simulink model "may21_slk"  (R2023b)
settings: Solver=VariableStepAuto  StartTime=0.0  StopTime=Tend_slk  RelTol=1e-3
values from neighbouring files (symbols this model uses):
  Ts_slk = 0.01    [may21_b_ml.m]    (also in may21_ml.m)
libraries: cstblocks x4, simulink x2
settings Model: Creator=Camilla  LastModifiedBy=Camilla

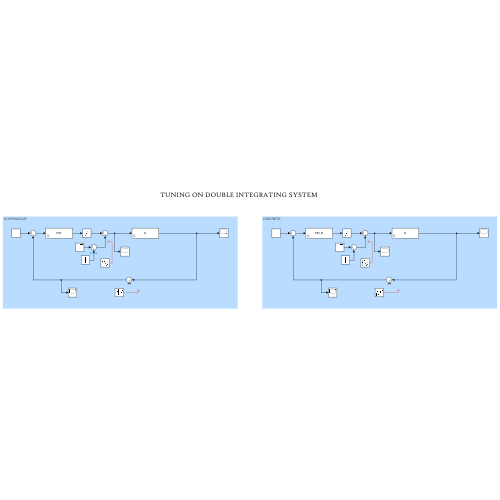
[thumbnail: Simulink's stored preview of the top-level diagram]
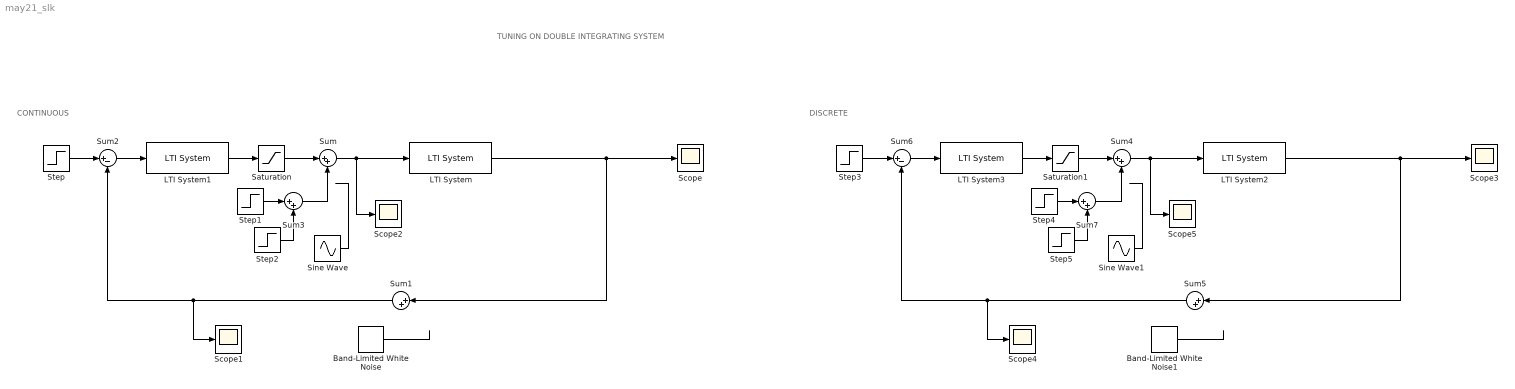
== system may21_slk ==
  note: TUNING ON DOUBLE INTEGRATING SYSTEM
  note: CONTINUOUS
  note: DISCRETE
  Band-Limited White Noise : simulink/Sources/Band-Limited White Noise  Cov=[0.0001]  Ts=0.05  seed=[23341]
  Band-Limited White Noise1 : simulink/Sources/Band-Limited White Noise  Cov=[0.0001]  Ts=0.05  seed=[23341]
  LTI System : cstblocks/LTI System  sys=G  IC=[]  PadeOrder=0
  LTI System1 : cstblocks/LTI System  sys=PID  IC=[]  PadeOrder=0
  LTI System2 : cstblocks/LTI System  sys=G  IC=[]  PadeOrder=0
  LTI System3 : cstblocks/LTI System  sys=PID_D  IC=[]  PadeOrder=0
  Saturation : Saturate  UpperLimit=1.2  LowerLimit=-1.2
  Saturation1 : Saturate  UpperLimit=1.2  LowerLimit=-1.2
  Scope{,1..5} (6 alike) : Scope
  Sine Wave : Sin  Amplitude=0.02  SampleTime=0
  Sine Wave1 : Sin  Amplitude=0.02  SampleTime=0
  Step : Step  Time=0  SampleTime=Ts_slk
  Step1 : Step  Time=200  After=0.2  SampleTime=Ts_slk
  Step2 : Step  Time=200.1  After=-0.2  SampleTime=Ts_slk
  Step3 : Step  Time=0  SampleTime=Ts_slk
  Step4 : Step  Time=200  After=0.2  SampleTime=Ts_slk
  Step5 : Step  Time=200.1  After=-0.2  SampleTime=Ts_slk
  Sum{,1,3..5,7} (6 alike) : Sum  Inputs=|++
  Sum2 : Sum  Inputs=|+-
  Sum6 : Sum  Inputs=|+-
  wires:
  Sum/1 -> Scope2/1, LTI System/1
  LTI System/1 -> Sum1/1, Scope/1
  Step/1 -> Sum2/1
  Sum1/1 -> Scope1/1, Sum2/2
  Sum2/1 -> LTI System1/1
  Sum3/1 -> Sum/2
  Step1/1 -> Sum3/1
  Step2/1 -> Sum3/2
  Saturation/1 -> Sum/1
  LTI System1/1 -> Saturation/1
  Band-Limited White Noise/1 -> ?
  Sine Wave/1 -> ?
  Sum7/1 -> Sum4/2
  Band-Limited White Noise1/1 -> ?
  Sum6/1 -> LTI System3/1
  LTI System3/1 -> Saturation1/1
  Sum4/1 -> Scope5/1, LTI System2/1
  Step3/1 -> Sum6/1
  Step5/1 -> Sum7/2
  Step4/1 -> Sum7/1
  Sine Wave1/1 -> ?
  Sum5/1 -> Scope4/1, Sum6/2
  Saturation1/1 -> Sum4/1
  LTI System2/1 -> Sum5/1, Scope3/1
